simulink model "Pulses__Input"  (Simulink 9.3)
settings: Solver=ode45  StartTime=0.0  StopTime=39  MaxStep=pi/1000  RelTol=1e-6  AbsTol=1e-8  EnableMultiTasking=on
InitFcn:
  | M=10; C=0.5; K=1000;
libraries: simulink x1
settings Model: Creator=David  LastModifiedBy=sulaymon.eshkabilov
settings SolverCC: AutoScaleAbsTol=off
settings DataIOCC: LimitDataPoints=on
settings OptimizationCC: ExpressionDepthLimit=2147483647
settings DebuggingCC: SolverPrmCheckMsg=warning  StateNameClashWarn=warning
settings GRTTargetCC: GeneratePreprocessorConditionals=Disable all

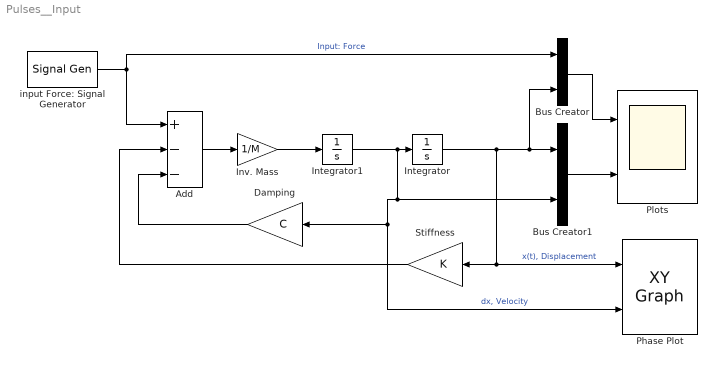
== system Pulses__Input ==
  Add : Sum  Inputs=+--
  Bus Creator : BusCreator  Inputs=2
  Bus Creator1 : BusCreator  Inputs=2
  Damping : Gain  Gain=C
  Integrator : Integrator
  Integrator1 : Integrator
  Inv. Mass : Gain  Gain=1/M
  Phase Plot : simulink/Sinks/XY Graph  xmin=-.8  xmax=.8  ymin=-8  ymax=8  st=-1
  Plots : Scope  NumInputPorts=2
  Stiffness : Gain  Gain=K
  input Force: Signal Generator : SignalGenerator  WaveForm=square  Amplitude=-100  Frequency=.5
  wires:
  Integrator1/1 -> Integrator/1, Bus Creator1/2, Phase Plot/2, Damping/1  "dx, Velocity"
  Inv. Mass/1 -> Integrator1/1
  Integrator/1 -> Bus Creator/2, Bus Creator1/1, Phase Plot/1, Stiffness/1  "x(t), Displacement"
  Damping/1 -> Add/3
  Stiffness/1 -> Add/2
  input Force: Signal Generator/1 -> Add/1, Bus Creator/1  "Input: Force"
  Add/1 -> Inv. Mass/1
  Bus Creator/1 -> Plots/1
  Bus Creator1/1 -> Plots/2
